simulink model "Tdof_robot_z"  (R2018a)
settings: Solver=ode4  StartTime=0.0  StopTime=10  FixedStep=1e-4  RelTol=1e-3
libraries: simulink x4, powerlib_meascontrol x2
settings Model: Creator=oussa  LastModifiedBy=oussa

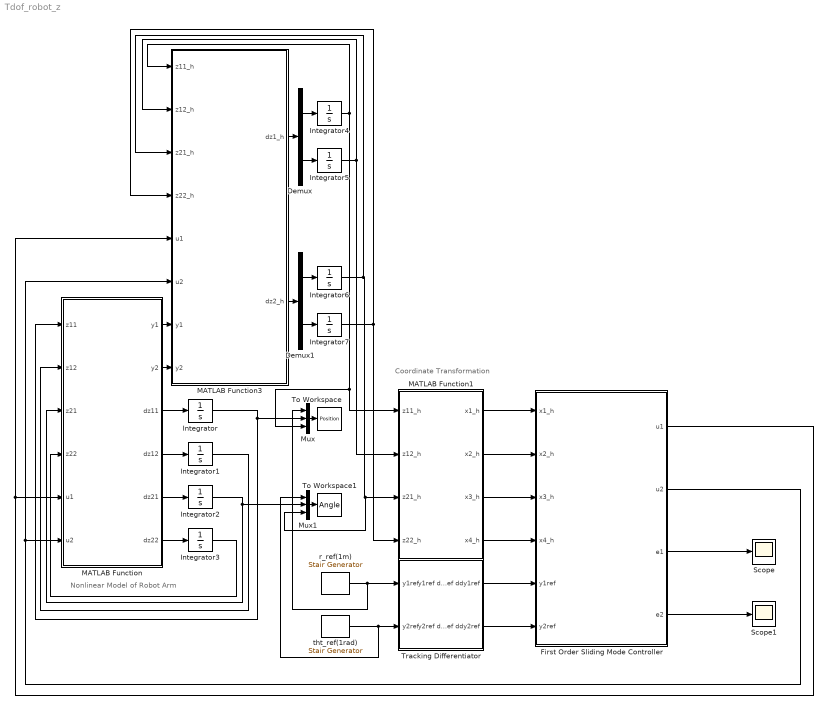
== system Tdof_robot_z ==
  note: Coordinate Transformation
  note: Nonlinear Model of Robot Arm
  Demux : Demux  Outputs=2
  Demux1 : Demux  Outputs=2
  First Order Sliding Mode Controller : MATLAB Function  TreatAsAtomicUnit=on
  Integrator : Integrator  InitialCondition=0.01
  Integrator1 : Integrator
  Integrator2 : Integrator
  Integrator3 : Integrator
  Integrator4 : Integrator  InitialCondition=0.3
  Integrator5 : Integrator  InitialCondition=0.01
  Integrator6 : Integrator  InitialCondition=0.4
  Integrator7 : Integrator  InitialCondition=0.01
  MATLAB Function : MATLAB Function  TreatAsAtomicUnit=on
  MATLAB Function1 : MATLAB Function  TreatAsAtomicUnit=on
  MATLAB Function3 : MATLAB Function  TreatAsAtomicUnit=on
  Mux : Mux  Inputs=3
  Mux1 : Mux  Inputs=3
  Scope : Scope
  Scope1 : Scope
  To Workspace : ToWorkspace  VariableName=Position  SampleTime=-1
  To Workspace1 : ToWorkspace  VariableName=Angle  SampleTime=-1
  Tracking Differentiator : Subsystem
  r_ref(1m) : powerlib_meascontrol/Pulse & Signal Generators/Stair Generator  t=[0, 1, 3, 6, 10]  e=[1, 0.5, 2.5, 2,1]  Ts=0
      settings: SourceProductName=Simscape Power Systems
  tht_ref(1rad) : powerlib_meascontrol/Pulse & Signal Generators/Stair Generator  t=[0, 2, 5, 8, 10]  e=[1, 1.5, 0.8, 1.7, 2]  Ts=0
      settings: SourceProductName=Simscape Power Systems
  wires:
  MATLAB Function/4(dz12) -> Integrator1/1
  MATLAB Function/5(dz21) -> Integrator2/1
  MATLAB Function/6(dz22) -> Integrator3/1
  Tracking Differentiator/1(y1ref dy1ref ddy1ref) -> First Order Sliding Mode Controller/5(y1ref)
  Tracking Differentiator/2(y2ref dy2ref ddy2ref) -> First Order Sliding Mode Controller/6(y2ref)
  MATLAB Function/1(y1) -> MATLAB Function3/7(y1)
  MATLAB Function/2(y2) -> MATLAB Function3/8(y2)
  MATLAB Function/3(dz11) -> Integrator/1
  Integrator1/1 -> MATLAB Function/2(z12)
  Integrator2/1 -> Mux1/2, MATLAB Function/3(z21)
  Integrator3/1 -> MATLAB Function/4(z22)
  First Order Sliding Mode Controller/3(e1) -> Scope/1
  First Order Sliding Mode Controller/4(e2) -> Scope1/1
  MATLAB Function1/1(x1_h) -> First Order Sliding Mode Controller/1(x1_h)
  MATLAB Function1/2(x2_h) -> First Order Sliding Mode Controller/2(x2_h)
  MATLAB Function1/3(x3_h) -> First Order Sliding Mode Controller/3(x3_h)
  MATLAB Function1/4(x4_h) -> First Order Sliding Mode Controller/4(x4_h)
  Integrator4/1 -> MATLAB Function3/1(z11_h), Mux/3, MATLAB Function1/1(z11_h)
  Integrator5/1 -> MATLAB Function1/2(z12_h), MATLAB Function3/2(z12_h)
  Integrator6/1 -> Mux1/3, MATLAB Function1/3(z21_h), MATLAB Function3/3(z21_h)
  Integrator7/1 -> MATLAB Function1/4(z22_h), MATLAB Function3/4(z22_h)
  MATLAB Function3/1(dz1_h) -> Demux/1
  Demux/1 -> Integrator4/1
  Demux/2 -> Integrator5/1
  MATLAB Function3/2(dz2_h) -> Demux1/1
  Demux1/1 -> Integrator6/1
  Demux1/2 -> Integrator7/1
  First Order Sliding Mode Controller/2(u2) -> MATLAB Function/6(u2), MATLAB Function3/6(u2)
  First Order Sliding Mode Controller/1(u1) -> MATLAB Function3/5(u1), MATLAB Function/5(u1)
  tht_ref(1rad)/1 -> Mux1/1, Tracking Differentiator/2(y2ref)
  Integrator/1 -> MATLAB Function/1(z11), Mux/2
  r_ref(1m)/1 -> Mux/1, Tracking Differentiator/1(y1ref)
  Mux/1 -> To Workspace/1
  Mux1/1 -> To Workspace1/1

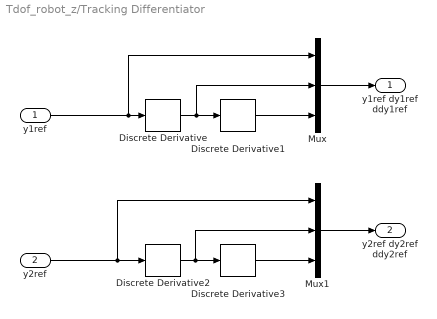
== system Tdof_robot_z/Tracking Differentiator ==
  y1ref : Inport
  y2ref : Inport  Port=2
  Discrete Derivative{,1..3} (4 alike) : simulink/Discrete/Discrete Derivative  gainval=eps  ICPrevScaledInput=0.0  OutMin=[]  OutMax=[]  OutDataType=fixdt(1, 16)  OutScaling=2^-10  DoSatur=off
  Mux : Mux  Inputs=3
  Mux1 : Mux  Inputs=3
  y1ref dy1ref ddy1ref : Outport
  y2ref dy2ref ddy2ref : Outport  Port=2
  wires:
  Discrete Derivative/1 -> Mux/2, Discrete Derivative1/1
  y1ref/1 -> Mux/1, Discrete Derivative/1
  Discrete Derivative2/1 -> Mux1/2, Discrete Derivative3/1
  y2ref/1 -> Mux1/1, Discrete Derivative2/1
  Discrete Derivative1/1 -> Mux/3
  Mux/1 -> y1ref dy1ref ddy1ref/1
  Discrete Derivative3/1 -> Mux1/3
  Mux1/1 -> y2ref dy2ref ddy2ref/1

== matlab function Tdof_robot_z/MATLAB Function1 ==
  data: z11_h input; x1_h output; z12_h input; z21_h input; z22_h input; x2_h output; x3_h output; x4_h output
function [x1_h,x2_h,x3_h,x4_h] = CTI(z11_h,z12_h,z21_h,z22_h)

x1_h = z11_h;
x2_h = z12_h;
x3_h = z21_h;
x4_h = z22_h;

== matlab function Tdof_robot_z/MATLAB Function ==
  data: y1 output; y2 output; z11 input; dz11 output; z12 input; z21 input; z22 input; u1 input; u2 input; dz12 output; dz21 output; dz22 output
function [y1,y2,dz11,dz12,dz21,dz22] = Tdof_robot_z(z11,z12,z21,z22,u1,u2)
g = 9.8; m = 1;
phi1 = [0;z11*z22^2-g*sin(z21)+u1/m];
phi2 = [0;1/z11^2*(-2*z11*z12*z22-g*z11*cos(z21)+u2/m)];

A1 = [0 1;0 0];
C1 = [1 0];
z1 = [z11;z12];
dz1 = A1*z1+phi1;
y1 = C1*z1;

A2 = [0 1;0 0];
C2 = [1 0];
z2 = [z21;z22];
dz2 = A2*z2+phi2;
y2 = C2*z2;

dz11 = dz1(1);
dz12 = dz1(2);
dz21 = dz2(1);
dz22 = dz2(2);
end

== matlab function Tdof_robot_z/First Order Sliding Mode Controller ==
  data: x1_h input; u1 output; x2_h input; x3_h input; x4_h input; y1ref input size=3; y2ref input size=3; u2 output; e1 output; e2 output
function [u1,u2,e1,e2] = FOSMC(x1_h,x2_h,x3_h,x4_h,y1ref,y2ref)
%% Manipulator Mass and Gravity
m = 1; g = 9.8;
%% Attractivity and Stability constants for sliding surface
k1 = 20; k2 = 20;
lambda1 = 20; lambda2 = 20;
y1 = x1_h;
y2 = x3_h;
dy1 = x2_h;
dy2 = x4_h;
dy1ref = y1ref(2);
dy2ref = y2ref(2);
ddy1ref = y1ref(3);
ddy2ref = y2ref(3);
%% Errors and their derivatives
e1 = y1-y1ref(1);
e2 = y2-y2ref(1);
de1 = dy1-dy1ref;
de2 = dy2-dy2ref;
%% Sliding surfaces
s1 = de1+lambda1*e1;
s2 = de2+lambda2*e2;
%% Control law : u = ueq+udisc
u1 = m*(-x1_h*x4_h^2+g*sin(x3_h)+ddy1ref-lambda1*de1-k1*sign(s1));
u2 = m*x1_h^2*(1/x1_h*(2*x2_h*x4_h+g*cos(x3_h))-lambda2*de2+ddy2ref-k2*sign(s2));
end

== matlab function Tdof_robot_z/MATLAB Function3 ==
  data: dz1_h output size=2; z11_h input; z12_h input; z21_h input; z22_h input; u1 input; u2 input; y1 input; y2 input; dz2_h output size=2
function [dz1_h, dz2_h] = High_gain_observer(z11_h,z12_h,z21_h,z22_h,u1,u2,y1,y2)
g = 9.8; m = 1;
phi1_h = [0;z11_h*z22_h^2-g*sin(z21_h)+u1/m];
phi2_h = [0;1/z11_h^2*(-2*z11_h*z12_h*z22_h-g*z11_h*cos(z21_h)+u2/m)];
teta = 10;
S1 = zeros(length(phi1_h),length(phi1_h));
S2 = zeros(length(phi2_h),length(phi2_h));
for i=1:length(phi1_h)
    for j=1:length(phi2_h)
        C = factorial(i+j-2)/(factorial(i+j-2-(j-1))*factorial(j-1));
        S1(i,j) = (-1)^(i+j)*C/(teta^(i+j-1));
        S2(i,j) = (-1)^(i+j)*C/(teta^(i+j-1));
    end
end
A1 = [0 1;0 0];
C1 = [1 0];
A2 = A1;
C2 = C1;
dz1_h = A1*[z11_h;z12_h]+phi1_h-inv(S1)*C1'*(C1*[z11_h;z12_h]-y1);
dz2_h = A2*[z21_h;z22_h]+phi2_h-inv(S2)*C2'*(C2*[z21_h;z22_h]-y2);

end
